simulink model "openloop_response_2020b"  (R2020b)
settings: Solver=ode15s  StartTime=0.0  StopTime=20  RelTol=1e-7  AbsTol=1e-7  EnableMultiTasking=on
values from neighbouring files (symbols this model uses):
  c_bar = 0.5    [main.m]
  cp = 0.239    [datacstr.m]    (also in main.m; pplane10b.m = get(ppdisp,'currentpoint'))
  DH = -5*10^4    (= -50000)    [datacstr.m]    (also in main.m)
  ER = 8750    [datacstr.m]    (also in main.m)
  ko = 7.2*10^10    (= 72000000000)    [datacstr.m]    (also in main.m)
  q = 100    [datacstr.m]    (also in main.m)
  r = 1000    [datacstr.m]    (also in main.m; pplane10b.m = abs(z))
  T_bar = 350    [main.m]
  Tf = 350    [datacstr.m]    (also in main.m)
  UA = 5*10^4    (= 50000)    [datacstr.m]    (also in main.m)
  V = 100    [datacstr.m]    (also in main.m)
undefined symbols (not defined in the file or in its folder): cstrfun
libraries: simulink x1
settings Model: ExtModeTrigMode=oneshot  ExtModeArmWhenConnect=off  Creator=scattolini  LastModifiedBy=annab
settings SolverCC: AutoScaleAbsTol=off
settings DataIOCC: SaveFormat=Array  SignalLoggingSaveFormat=ModelDataLogs  ReturnWorkspaceOutputs=off  SignalLoggingName=sigsOut
settings OptimizationCC: BlockReduction=off  BooleanDataType=off  DefaultParameterBehavior=Inlined  BufferReuse=off  ExpressionDepthLimit=2147483647  InitFltsAndDblsToZero=on  LifeSpan=inf
settings DebuggingCC: SaveWithParameterizedLinksMsg=none  UnderspecifiedInitializationDetection=Classic  MergeDetectMultiDrivingBlocksExec=none  SignalResolutionControl=TryResolveAllWithWarning  MultiTaskDSMMsg=warning  MultiTaskCondExecSysMsg=none  FcnCallInpInsideContextMsg=warning  StateNameClashWarn=warning  SFUnexpectedBacktrackingDiag=warning  SFNoUnconditionalDefaultTransitionDiag=warning  SFExecutionAtInitializationDiag=none  ArithmeticOperatorsInVariantConditions=warning
settings HardwareCC: ProdBitPerPointer=32  ProdBitPerSizeT=32  ProdBitPerPtrDiffT=32  ProdLargestAtomicFloat=None  ProdIntDivRoundTo=Undefined  ProdEndianess=Unspecified  ProdWordSize=32  ProdHWDeviceType=32-bit Generic  TargetUnknown=on
settings ModelReferenceCC: PropagateSignalLabelsOutOfModel=off
settings SFSimCC: SimUseLocalCustomCode=off  CustomCodeUndefinedFunction=UseInterfaceOnly
settings RTWCC: RTWUseLocalCustomCode=off
settings CodeAppCC: StateflowObjectComments=on
settings GRTTargetCC: TargetFcnLib=ansi_tfl_tmw.mat  TargetLangStandard=C89/C90 (ANSI)  CombineOutputUpdateFcns=off  GRTInterface=on
settings ConfigComp: CovMetricSettings=dw  CovSaveCumulativeToWorkspaceVar=on  CovSaveSingleToWorkspaceVar=on  CovExternalEMLEnable=off  CovSFcnEnable=off

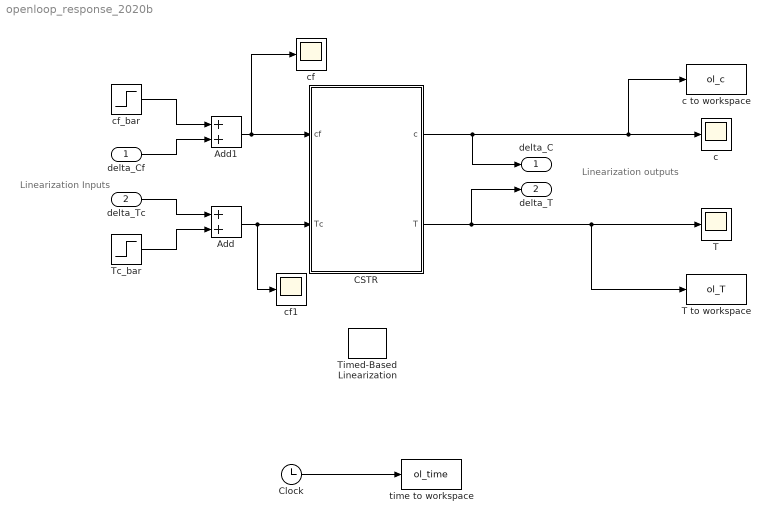
== system openloop_response_2020b ==
  note: Linearization
      | Inputs
  note: Linearization
      | outputs
  delta_Cf : Inport
  delta_Tc : Inport  Port=2
  Add : Sum
  Add1 : Sum
  CSTR : Subsystem
  Clock : Clock
  T : Scope
  "T to workspace " : ToWorkspace  VariableName=ol_T  SampleTime=-1
  Tc_bar : Step  Time=0  Before=300  After=300  SampleTime=0
  Timed-Based Linearization : simulink/Model-Wide Utilities/Timed-Based Linearization  LinearizationTime=0.5  SampleTime=0
      settings: SourceProductBaseCode=SL
  c : Scope
  "c to workspace " : ToWorkspace  VariableName=ol_c  SampleTime=-1
  cf : Scope
  cf1 : Scope
  cf_bar : Step  Time=0  Before=1  SampleTime=0
  time to workspace : ToWorkspace  VariableName=ol_time  SampleTime=-1
  delta_C : Outport
  delta_T : Outport  Port=2
  wires:
  Clock/1 -> time to workspace/1
  CSTR/1(c) -> delta_C/1, c/1, "c to workspace "/1
  CSTR/2(T) -> delta_T/1, T/1, "T to workspace "/1
  Add/1 -> cf1/1, CSTR/2(Tc)
  Add1/1 -> cf/1, CSTR/1(cf)
  Tc_bar/1 -> Add/2
  cf_bar/1 -> Add1/1
  delta_Cf/1 -> Add1/2
  delta_Tc/1 -> Add/1

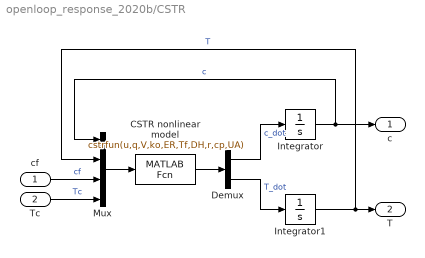
== system openloop_response_2020b/CSTR ==
  cf : Inport
  Tc : Inport  Port=2
  CSTR nonlinear model : MATLABFcn  MATLABFcn=cstrfun(u,q,V,ko,ER,Tf,DH,r,cp,UA)
  Demux : Demux  Outputs=2
      settings: DisplayOption=none
  Integrator : Integrator  InitialCondition=c_bar
  Integrator1 : Integrator  InitialCondition=T_bar
  Mux : Mux
  c : Outport
  T : Outport  Port=2
  wires:
  Mux/1 -> CSTR nonlinear model/1
  CSTR nonlinear model/1 -> Demux/1
  Demux/1 -> Integrator/1  "c_dot"
  Demux/2 -> Integrator1/1  "T_dot"
  Integrator1/1 -> Mux/2, T/1  "T"
  Integrator/1 -> Mux/1, c/1  "c"
  cf/1 -> Mux/3  "cf"
  Tc/1 -> Mux/4  "Tc"
